simulink model "casper_sim_phase0"  (R2025b)
settings: Solver=FixedStepDiscrete  StartTime=-5  StopTime=5  FixedStep=1e-3  RelTol=1e-3
InitFcn:
  | casper_prelaunch_pad_truth_ts(5.0);
undefined symbols (not defined in the file or in its folder): Estimator
libraries: imu_block_visual x2, baro_block_visual x1, gps_block_visual x1, mag_block_visual x1
settings Model: Creator=Ashwin  LastModifiedBy=Ashwin
settings DebuggingCC: InheritedTsInSrcMsg=none

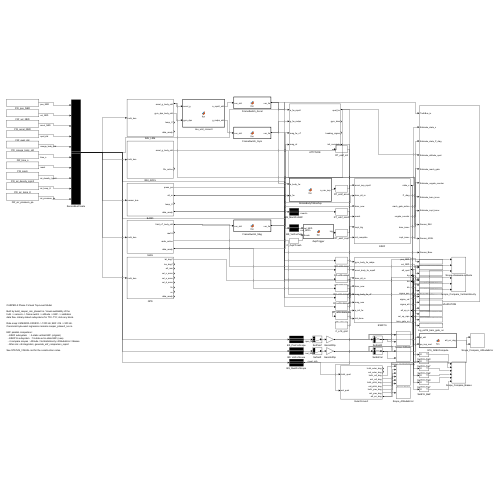
[thumbnail: Simulink's stored preview of the top-level diagram]
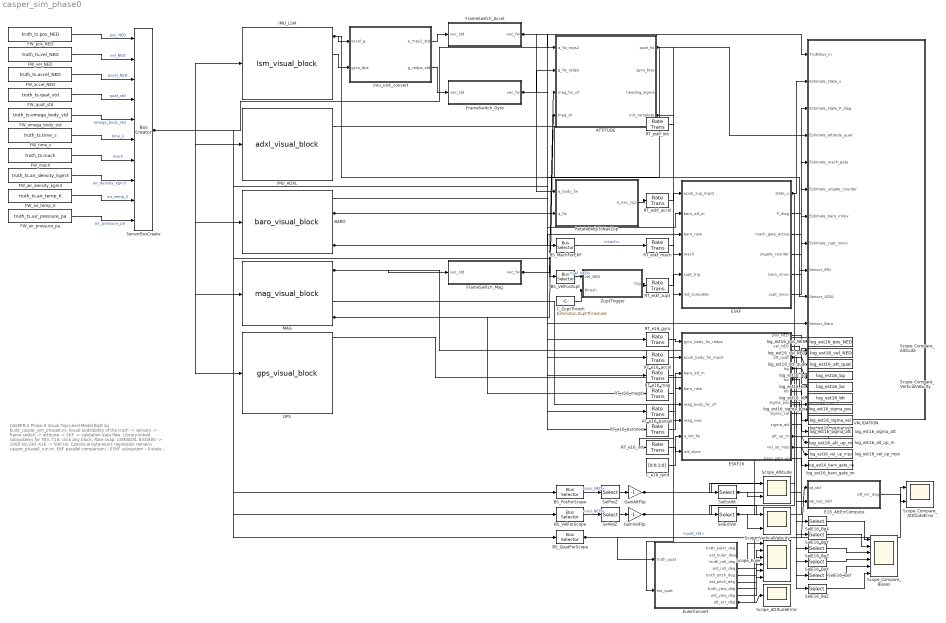
== system casper_sim_phase0 ==
  note: CASPER-2 Phase 0 Visual Top-Level Model
      |
      | Built by build_casper_sim_phase0.m. Visual auditability of the
      | truth -> sensors -> frame switch -> attitude -> EKF -> validation
      | data flow. Library-linked subsystems for T03..T10; click any block.
      |
      | Rate snap: LSM/ADXL 833/800 -> 1000 Hz; EKF 416 -> 500 Hz.
      | Canonical byte-exact regression remains casper_phase0_run.m.
      |
      | EKF parallel comparison:
      |   - ESKF subsystem    : 4-state vertical EKF (original)
      |   - ESKF16 subsystem  : 16-state error-state EKF (new)
      |   - 4 compare scopes  : Altitude / VerticalVelocity / AttitudeError / Biases
      |   - After sim: cd integration; generate_ekf_comparison_report
      |
      | See STATUS_VISUAL.md for the construction notes.
  ATTITUDE : Subsystem
  BARO : baro_block_visual/baro_visual_block  SystemSampleTime=-1  VariantActivationTime=update diagram  EmptyChoice=off  PassThrough=off  PassThroughVariantControl=(default)  EmptyChoiceVariantControl=(default)  AllowFlexibleInterface=on  Latency=0  AutoFrameSizeCalculation=off
  BS_MachForEKF : BusSelector  OutputSignals=mach
  BS_PosForScope : BusSelector  OutputSignals=pos_NED
  BS_QuatForScope : BusSelector  OutputSignals=quat_std
  BS_VelForScope : BusSelector  OutputSignals=vel_NED
  BS_VelForZupt : BusSelector  OutputSignals=vel_NED
  C_ZuptThresh : Constant  Value=Estimator.ZuptThreshold  SampleTime=-1
  C_e16_qinit : Constant  Value=[0;0;1;0]  SampleTime=-1
  E16_AttErrCompute : MATLAB Function  TreatAsAtomicUnit=on
  ESKF : Subsystem
  ESKF16 : Subsystem
  EulerConvert : Subsystem
  FW_accel_NED : FromWorkspace  VariableName=truth_ts.accel_NED  SampleTime=-1  ZeroCross=off  OutputAfterFinalValue=Holding final value
  FW_air_density_kgm3 : FromWorkspace  VariableName=truth_ts.air_density_kgm3  SampleTime=-1  ZeroCross=off  OutputAfterFinalValue=Holding final value
  FW_air_pressure_pa : FromWorkspace  VariableName=truth_ts.air_pressure_pa  SampleTime=-1  ZeroCross=off  OutputAfterFinalValue=Holding final value
  FW_air_temp_K : FromWorkspace  VariableName=truth_ts.air_temp_K  SampleTime=-1  ZeroCross=off  OutputAfterFinalValue=Holding final value
  FW_mach : FromWorkspace  VariableName=truth_ts.mach  SampleTime=-1  ZeroCross=off  OutputAfterFinalValue=Holding final value
  FW_omega_body_std : FromWorkspace  VariableName=truth_ts.omega_body_std  SampleTime=-1  ZeroCross=off  OutputAfterFinalValue=Holding final value
  FW_pos_NED : FromWorkspace  VariableName=truth_ts.pos_NED  SampleTime=-1  ZeroCross=off  OutputAfterFinalValue=Holding final value
  FW_quat_std : FromWorkspace  VariableName=truth_ts.quat_std  SampleTime=-1  ZeroCross=off  OutputAfterFinalValue=Holding final value
  FW_time_s : FromWorkspace  VariableName=truth_ts.time_s  SampleTime=-1  ZeroCross=off  OutputAfterFinalValue=Holding final value
  FW_vel_NED : FromWorkspace  VariableName=truth_ts.vel_NED  SampleTime=-1  ZeroCross=off  OutputAfterFinalValue=Holding final value
  FrameSwitch_Accel : MATLAB Function  TreatAsAtomicUnit=on
  FrameSwitch_Gyro : MATLAB Function  TreatAsAtomicUnit=on
  FrameSwitch_Mag : MATLAB Function  TreatAsAtomicUnit=on
  GPS : gps_block_visual/gps_visual_block  SystemSampleTime=-1  VariantActivationTime=update diagram  EmptyChoice=off  PassThrough=off  PassThroughVariantControl=(default)  EmptyChoiceVariantControl=(default)  AllowFlexibleInterface=on  Latency=0  AutoFrameSizeCalculation=off
  GainAltFlip : Gain  Gain=-1
  GainVelFlip : Gain  Gain=-1
  IMU_ADXL : imu_block_visual/adxl_visual_block  SystemSampleTime=-1  VariantActivationTime=update diagram  EmptyChoice=off  PassThrough=off  PassThroughVariantControl=(default)  EmptyChoiceVariantControl=(default)  AllowFlexibleInterface=on  Latency=0  AutoFrameSizeCalculation=off
  IMU_LSM : imu_block_visual/lsm_visual_block  SystemSampleTime=-1  VariantActivationTime=update diagram  EmptyChoice=off  PassThrough=off  PassThroughVariantControl=(default)  EmptyChoiceVariantControl=(default)  AllowFlexibleInterface=on  Latency=0  AutoFrameSizeCalculation=off
  MAG : mag_block_visual/mag_visual_block  SystemSampleTime=-1  VariantActivationTime=update diagram  EmptyChoice=off  PassThrough=off  PassThroughVariantControl=(default)  EmptyChoiceVariantControl=(default)  AllowFlexibleInterface=on  Latency=0  AutoFrameSizeCalculation=off
  RT_e16_accel : RateTransition  OutPortSampleTime=2e-3
  RT_e16_baroalt : RateTransition  OutPortSampleTime=2e-3
  RT_e16_baronew : RateTransition  OutPortSampleTime=2e-3
  RT_e16_gyro : RateTransition  OutPortSampleTime=2e-3
  RT_e16_init : RateTransition  OutPortSampleTime=2e-3
  RT_e16_mag : RateTransition  OutPortSampleTime=2e-3
  RT_e16_magdr : RateTransition  OutPortSampleTime=2e-3
  RT_eskf_accel : RateTransition  OutPortSampleTime=2e-3
  RT_eskf_init : RateTransition  OutPortSampleTime=2e-3
  RT_eskf_mach : RateTransition  OutPortSampleTime=2e-3
  RT_eskf_zupt : RateTransition  OutPortSampleTime=2e-3
  RotateBodyToNavZup : MATLAB Function  TreatAsAtomicUnit=on
  Scope_Altitude : Scope  NumInputPorts=2
      settings: Title=Altitude - truth vs estimate [m]
  Scope_AttitudeError : Scope
      settings: Title=Attitude error magnitude [deg]
  Scope_Compare_Altitude : Scope  NumInputPorts=3
      settings: Title=Altitude compare - truth vs 4-state vs 16-state [m]
  Scope_Compare_AttitudeError : Scope  NumInputPorts=2
      settings: Title=Attitude error compare - 4-state vs 16-state [deg]
  Scope_Compare_Biases : Scope  NumInputPorts=6
      settings: Title=16-state biases - gyro xyz (rad/s) + accel xyz (m/s^2)
  Scope_Compare_VerticalVelocity : Scope  NumInputPorts=3
      settings: Title=Vertical velocity compare - truth vs 4-state vs 16-state [m/s]
  Scope_Euler : Scope  NumInputPorts=6
      settings: Title=Orientation Euler - truth vs estimate [deg]
  Scope_VerticalVelocity : Scope  NumInputPorts=2
      settings: Title=Vertical velocity - truth vs estimate [m/s]
  SelE16_BaX : Selector  InputPortWidth=3  IndexOptions=Index vector (dialog)  Indices=1  OutputSizes=1
  SelE16_BaY : Selector  InputPortWidth=3  IndexOptions=Index vector (dialog)  Indices=2  OutputSizes=1
  SelE16_BaZ : Selector  InputPortWidth=3  IndexOptions=Index vector (dialog)  Indices=3  OutputSizes=1
  SelE16_BgX : Selector  InputPortWidth=3  IndexOptions=Index vector (dialog)  Indices=1  OutputSizes=1
  SelE16_BgY : Selector  InputPortWidth=3  IndexOptions=Index vector (dialog)  Indices=2  OutputSizes=1
  SelE16_BgZ : Selector  InputPortWidth=3  IndexOptions=Index vector (dialog)  Indices=3  OutputSizes=1
  SelEstAlt : Selector  InputPortWidth=4  IndexOptions=Index vector (dialog)  Indices=1  OutputSizes=1
  SelEstVel : Selector  InputPortWidth=4  IndexOptions=Index vector (dialog)  Indices=2  OutputSizes=1
  SelPosZ : Selector  InputPortWidth=3  IndexOptions=Index vector (dialog)  Indices=3  OutputSizes=1
  SelVelZ : Selector  InputPortWidth=3  IndexOptions=Index vector (dialog)  Indices=3  OutputSizes=1
  SensorBusCreate : BusCreator  Inputs=10  OutDataTypeStr=Bus: SensorInputBus  NonVirtualBus=on
  VALIDATION : Subsystem
  ZuptTrigger : MATLAB Function  TreatAsAtomicUnit=on
  imu_unit_convert : MATLAB Function  TreatAsAtomicUnit=on
  log_est16_alt_up_m : ToWorkspace  VariableName=log_est16_alt_up_m  SaveFormat=Structure With Time  SampleTime=-1
  log_est16_att_quat : ToWorkspace  VariableName=log_est16_att_quat  SaveFormat=Structure With Time  SampleTime=-1
  log_est16_ba : ToWorkspace  VariableName=log_est16_ba  SaveFormat=Structure With Time  SampleTime=-1
  log_est16_baro_gate_on : ToWorkspace  VariableName=log_est16_baro_gate_on  SaveFormat=Structure With Time  SampleTime=-1
  log_est16_bb : ToWorkspace  VariableName=log_est16_bb  SaveFormat=Structure With Time  SampleTime=-1
  log_est16_bg : ToWorkspace  VariableName=log_est16_bg  SaveFormat=Structure With Time  SampleTime=-1
  log_est16_pos_NED : ToWorkspace  VariableName=log_est16_pos_NED  SaveFormat=Structure With Time  SampleTime=-1
  log_est16_sigma_att : ToWorkspace  VariableName=log_est16_sigma_att  SaveFormat=Structure With Time  SampleTime=-1
  log_est16_sigma_pos : ToWorkspace  VariableName=log_est16_sigma_pos  SaveFormat=Structure With Time  SampleTime=-1
  log_est16_sigma_vel : ToWorkspace  VariableName=log_est16_sigma_vel  SaveFormat=Structure With Time  SampleTime=-1
  log_est16_vel_NED : ToWorkspace  VariableName=log_est16_vel_NED  SaveFormat=Structure With Time  SampleTime=-1
  log_est16_vel_up_mps : ToWorkspace  VariableName=log_est16_vel_up_mps  SaveFormat=Structure With Time  SampleTime=-1
  wires:
  FW_pos_NED/1 -> SensorBusCreate/1  "pos_NED"
  FW_vel_NED/1 -> SensorBusCreate/2  "vel_NED"
  FW_accel_NED/1 -> SensorBusCreate/3  "accel_NED"
  FW_quat_std/1 -> SensorBusCreate/4  "quat_std"
  FW_omega_body_std/1 -> SensorBusCreate/5  "omega_body_std"
  FW_time_s/1 -> SensorBusCreate/6  "time_s"
  FW_mach/1 -> SensorBusCreate/7  "mach"
  FW_air_density_kgm3/1 -> SensorBusCreate/8  "air_density_kgm3"
  FW_air_temp_K/1 -> SensorBusCreate/9  "air_temp_K"
  FW_air_pressure_pa/1 -> SensorBusCreate/10  "air_pressure_pa"
  SensorBusCreate/1 -> IMU_LSM/1, IMU_ADXL/1, BARO/1, MAG/1, GPS/1, BS_MachForEKF/1, BS_VelForZupt/1, VALIDATION/1(TruthBus_in), BS_PosForScope/1, BS_VelForScope/1, BS_QuatForScope/1
  IMU_LSM/1 -> imu_unit_convert/1(accel_g), VALIDATION/9(Sensor_IMU)
  IMU_LSM/2 -> imu_unit_convert/2(gyro_dps)
  imu_unit_convert/1(a_mps2_std) -> FrameSwitch_Accel/1(vec_std)
  imu_unit_convert/2(g_radps_std) -> FrameSwitch_Gyro/1(vec_std)
  MAG/1 -> FrameSwitch_Mag/1(vec_std), VALIDATION/12(Sensor_Mag)
  FrameSwitch_Accel/1(vec_fw) -> ATTITUDE/1(a_fw_mps2), RotateBodyToNavZup/1(a_body_fw), RT_e16_accel/1
  FrameSwitch_Gyro/1(vec_fw) -> ATTITUDE/2(g_fw_radps), RT_e16_gyro/1
  FrameSwitch_Mag/1(vec_fw) -> ATTITUDE/3(mag_fw_uT), RT_e16_mag/1
  MAG/4 -> ATTITUDE/4(mag_dr), RT_e16_magdr/1
  ATTITUDE/1(quat_fw) -> RotateBodyToNavZup/2(q_fw), VALIDATION/4(Estimate_attitude_quat), EulerConvert/2(est_quat)
  RotateBodyToNavZup/1(a_nav_zup) -> RT_eskf_accel/1
  BS_MachForEKF/1 -> RT_eskf_mach/1  "<mach>"
  BS_VelForZupt/1 -> ZuptTrigger/1(vel_NED)  "<vel_NED>"
  C_ZuptThresh/1 -> ZuptTrigger/2(thresh)
  ZuptTrigger/1(trig) -> RT_eskf_zupt/1
  ATTITUDE/4(init_complete) -> RT_eskf_init/1, RT_e16_init/1
  RT_eskf_accel/1 -> ESKF/1(accel_zup_mps2)
  BARO/2 -> ESKF/2(baro_alt_m), RT_e16_baroalt/1
  BARO/4 -> ESKF/3(baro_new), RT_e16_baronew/1
  RT_eskf_mach/1 -> ESKF/4(mach)
  RT_eskf_zupt/1 -> ESKF/5(zupt_trig)
  RT_eskf_init/1 -> ESKF/6(init_complete)
  ESKF/1(state_x) -> VALIDATION/2(Estimate_state_x), SelEstAlt/1, SelEstVel/1
  ESKF/2(P_diag) -> VALIDATION/3(Estimate_state_P_diag)
  ESKF/3(mach_gate_active) -> VALIDATION/5(Estimate_mach_gate)
  ESKF/4(ungate_counter) -> VALIDATION/6(Estimate_ungate_counter)
  ESKF/5(baro_innov) -> VALIDATION/7(Estimate_baro_innov)
  ESKF/6(zupt_innov) -> VALIDATION/8(Estimate_zupt_innov)
  IMU_ADXL/1 -> VALIDATION/10(Sensor_ADXL)
  BARO/1 -> VALIDATION/11(Sensor_Baro)
  GPS/1 -> VALIDATION/13(Sensor_GPS)
  MAG/3 -> VALIDATION/14(RadioTX_active)
  BS_PosForScope/1 -> SelPosZ/1  "<pos_NED>"
  SelPosZ/1 -> GainAltFlip/1
  BS_VelForScope/1 -> SelVelZ/1  "<vel_NED>"
  SelVelZ/1 -> GainVelFlip/1
  BS_QuatForScope/1 -> EulerConvert/1(truth_quat), E16_AttErrCompute/1(qt_std)  "<quat_std>"
  GainAltFlip/1 -> Scope_Altitude/1, Scope_Compare_Altitude/1
  SelEstAlt/1 -> Scope_Altitude/2, Scope_Compare_Altitude/2
  GainVelFlip/1 -> Scope_VerticalVelocity/1, Scope_Compare_VerticalVelocity/1
  SelEstVel/1 -> Scope_VerticalVelocity/2, Scope_Compare_VerticalVelocity/2
  EulerConvert/3(truth_roll_deg) -> Scope_Euler/1
  EulerConvert/4(est_roll_deg) -> Scope_Euler/2
  EulerConvert/5(truth_pitch_deg) -> Scope_Euler/3
  EulerConvert/6(est_pitch_deg) -> Scope_Euler/4
  EulerConvert/7(truth_yaw_deg) -> Scope_Euler/5
  EulerConvert/8(est_yaw_deg) -> Scope_Euler/6
  EulerConvert/9(att_err_deg) -> Scope_AttitudeError/1, Scope_Compare_AttitudeError/1
  RT_e16_gyro/1 -> ESKF16/1(gyro_body_fw_radps)
  RT_e16_accel/1 -> ESKF16/2(accel_body_fw_mps2)
  RT_e16_baroalt/1 -> ESKF16/3(baro_alt_m)
  RT_e16_baronew/1 -> ESKF16/4(baro_new)
  RT_e16_mag/1 -> ESKF16/5(mag_body_fw_uT)
  RT_e16_magdr/1 -> ESKF16/6(mag_new)
  C_e16_qinit/1 -> ESKF16/7(q_init_fw)
  RT_e16_init/1 -> ESKF16/8(init_done)
  ESKF16/1(pos_NED) -> log_est16_pos_NED/1
  ESKF16/2(vel_NED) -> log_est16_vel_NED/1
  ESKF16/3(att_quat) -> log_est16_att_quat/1, E16_AttErrCompute/2(qe_zup_ned)
  ESKF16/4(bg) -> log_est16_bg/1, SelE16_BgX/1, SelE16_BgY/1, SelE16_BgZ/1
  ESKF16/5(ba) -> log_est16_ba/1, SelE16_BaX/1, SelE16_BaY/1, SelE16_BaZ/1
  ESKF16/6(bb) -> log_est16_bb/1
  ESKF16/7(sigma_pos) -> log_est16_sigma_pos/1
  ESKF16/8(sigma_vel) -> log_est16_sigma_vel/1
  ESKF16/9(sigma_att) -> log_est16_sigma_att/1
  ESKF16/10(alt_up_m) -> log_est16_alt_up_m/1, Scope_Compare_Altitude/3
  ESKF16/11(vel_up_mps) -> log_est16_vel_up_mps/1, Scope_Compare_VerticalVelocity/3
  ESKF16/12(baro_gate_on) -> log_est16_baro_gate_on/1
  E16_AttErrCompute/1(att_err_deg) -> Scope_Compare_AttitudeError/2
  SelE16_BgX/1 -> Scope_Compare_Biases/1
  SelE16_BgY/1 -> Scope_Compare_Biases/2
  SelE16_BgZ/1 -> Scope_Compare_Biases/3
  SelE16_BaX/1 -> Scope_Compare_Biases/4
  SelE16_BaY/1 -> Scope_Compare_Biases/5
  SelE16_BaZ/1 -> Scope_Compare_Biases/6

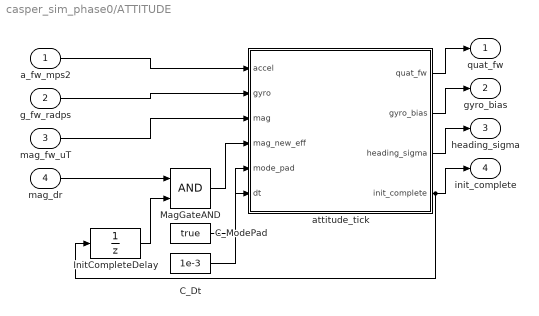
== system casper_sim_phase0/ATTITUDE ==
  a_fw_mps2 : Inport
  g_fw_radps : Inport  Port=2
  mag_fw_uT : Inport  Port=3
  mag_dr : Inport  Port=4
  C_Dt : Constant  Value=1e-3  SampleTime=-1
  C_ModePad : Constant  Value=true  OutDataTypeStr=boolean  SampleTime=-1
  InitCompleteDelay : UnitDelay  SampleTime=-1  HasFrameUpgradeWarning=on
  MagGateAND : Logic  AllPortsSameDT=off  OutDataTypeStr=boolean
  attitude_tick : MATLAB Function  TreatAsAtomicUnit=on
  quat_fw : Outport
  gyro_bias : Outport  Port=2
  heading_sigma : Outport  Port=3
  init_complete : Outport  Port=4
  wires:
  mag_dr/1 -> MagGateAND/1
  InitCompleteDelay/1 -> MagGateAND/2
  a_fw_mps2/1 -> attitude_tick/1(accel)
  g_fw_radps/1 -> attitude_tick/2(gyro)
  mag_fw_uT/1 -> attitude_tick/3(mag)
  MagGateAND/1 -> attitude_tick/4(mag_new_eff)
  C_ModePad/1 -> attitude_tick/5(mode_pad)
  C_Dt/1 -> attitude_tick/6(dt)
  attitude_tick/4(init_complete) -> InitCompleteDelay/1, init_complete/1
  attitude_tick/1(quat_fw) -> quat_fw/1
  attitude_tick/2(gyro_bias) -> gyro_bias/1
  attitude_tick/3(heading_sigma) -> heading_sigma/1

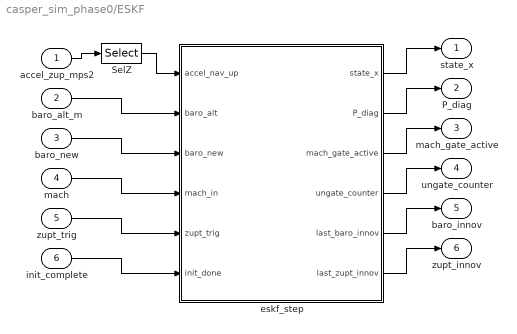
== system casper_sim_phase0/ESKF ==
  accel_zup_mps2 : Inport
  baro_alt_m : Inport  Port=2
  baro_new : Inport  Port=3
  mach : Inport  Port=4
  zupt_trig : Inport  Port=5
  init_complete : Inport  Port=6
  SelZ : Selector  InputPortWidth=3  IndexOptions=Index vector (dialog)  Indices=3  OutputSizes=1
  eskf_step : MATLAB Function  TreatAsAtomicUnit=on
  state_x : Outport
  P_diag : Outport  Port=2
  mach_gate_active : Outport  Port=3
  ungate_counter : Outport  Port=4
  baro_innov : Outport  Port=5
  zupt_innov : Outport  Port=6
  wires:
  accel_zup_mps2/1 -> SelZ/1
  SelZ/1 -> eskf_step/1(accel_nav_up)
  baro_alt_m/1 -> eskf_step/2(baro_alt)
  baro_new/1 -> eskf_step/3(baro_new)
  mach/1 -> eskf_step/4(mach_in)
  zupt_trig/1 -> eskf_step/5(zupt_trig)
  init_complete/1 -> eskf_step/6(init_done)
  eskf_step/1(state_x) -> state_x/1
  eskf_step/2(P_diag) -> P_diag/1
  eskf_step/3(mach_gate_active) -> mach_gate_active/1
  eskf_step/4(ungate_counter) -> ungate_counter/1
  eskf_step/5(last_baro_innov) -> baro_innov/1
  eskf_step/6(last_zupt_innov) -> zupt_innov/1

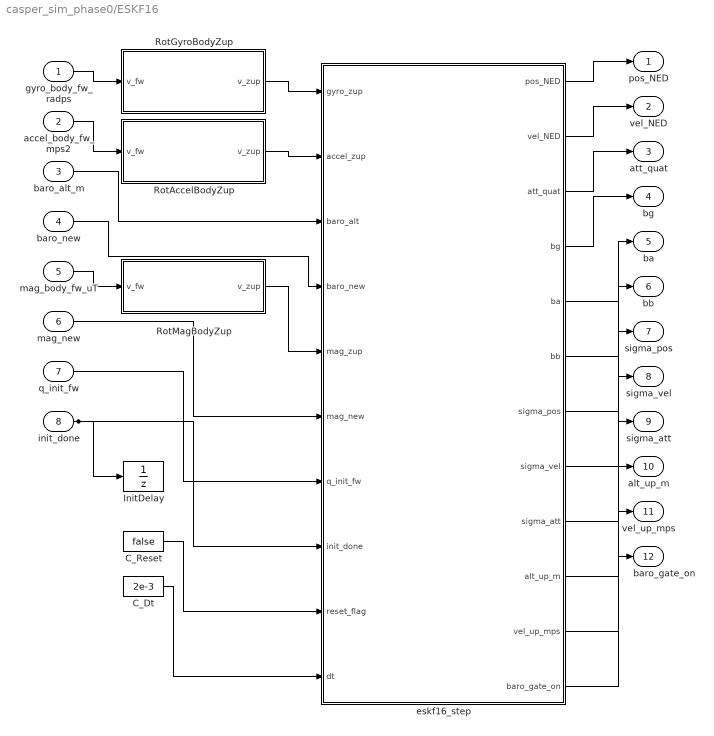
== system casper_sim_phase0/ESKF16 ==
  gyro_body_fw_radps : Inport
  accel_body_fw_mps2 : Inport  Port=2
  baro_alt_m : Inport  Port=3
  baro_new : Inport  Port=4
  mag_body_fw_uT : Inport  Port=5
  mag_new : Inport  Port=6
  q_init_fw : Inport  Port=7
  init_done : Inport  Port=8
  C_Dt : Constant  Value=2e-3  SampleTime=-1
  C_Reset : Constant  Value=false  OutDataTypeStr=boolean  SampleTime=-1
  InitDelay : UnitDelay  SampleTime=-1  HasFrameUpgradeWarning=on
  RotAccelBodyZup : MATLAB Function  TreatAsAtomicUnit=on
  RotGyroBodyZup : MATLAB Function  TreatAsAtomicUnit=on
  RotMagBodyZup : MATLAB Function  TreatAsAtomicUnit=on
  eskf16_step : MATLAB Function  TreatAsAtomicUnit=on
  pos_NED : Outport
  vel_NED : Outport  Port=2
  att_quat : Outport  Port=3
  bg : Outport  Port=4
  ba : Outport  Port=5
  bb : Outport  Port=6
  sigma_pos : Outport  Port=7
  sigma_vel : Outport  Port=8
  sigma_att : Outport  Port=9
  alt_up_m : Outport  Port=10
  vel_up_mps : Outport  Port=11
  baro_gate_on : Outport  Port=12
  wires:
  eskf16_step/12(baro_gate_on) -> baro_gate_on/1
  eskf16_step/11(vel_up_mps) -> vel_up_mps/1
  eskf16_step/10(alt_up_m) -> alt_up_m/1
  eskf16_step/9(sigma_att) -> sigma_att/1
  eskf16_step/8(sigma_vel) -> sigma_vel/1
  eskf16_step/7(sigma_pos) -> sigma_pos/1
  eskf16_step/6(bb) -> bb/1
  eskf16_step/5(ba) -> ba/1
  eskf16_step/4(bg) -> bg/1
  eskf16_step/3(att_quat) -> att_quat/1
  eskf16_step/2(vel_NED) -> vel_NED/1
  eskf16_step/1(pos_NED) -> pos_NED/1
  C_Dt/1 -> eskf16_step/10(dt)
  C_Reset/1 -> eskf16_step/9(reset_flag)
  q_init_fw/1 -> eskf16_step/7(q_init_fw)
  mag_new/1 -> eskf16_step/6(mag_new)
  RotMagBodyZup/1(v_zup) -> eskf16_step/5(mag_zup)
  baro_new/1 -> eskf16_step/4(baro_new)
  baro_alt_m/1 -> eskf16_step/3(baro_alt)
  RotAccelBodyZup/1(v_zup) -> eskf16_step/2(accel_zup)
  RotGyroBodyZup/1(v_zup) -> eskf16_step/1(gyro_zup)
  init_done/1 -> eskf16_step/8(init_done), InitDelay/1
  mag_body_fw_uT/1 -> RotMagBodyZup/1(v_fw)
  accel_body_fw_mps2/1 -> RotAccelBodyZup/1(v_fw)
  gyro_body_fw_radps/1 -> RotGyroBodyZup/1(v_fw)

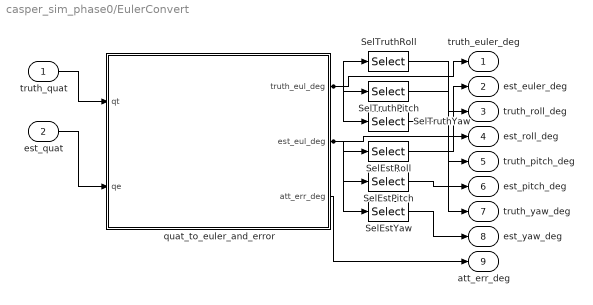
== system casper_sim_phase0/EulerConvert ==
  truth_quat : Inport
  est_quat : Inport  Port=2
  SelEstPitch : Selector  InputPortWidth=3  IndexOptions=Index vector (dialog)  Indices=2  OutputSizes=1
  SelEstRoll : Selector  InputPortWidth=3  IndexOptions=Index vector (dialog)  Indices=1  OutputSizes=1
  SelEstYaw : Selector  InputPortWidth=3  IndexOptions=Index vector (dialog)  Indices=3  OutputSizes=1
  SelTruthPitch : Selector  InputPortWidth=3  IndexOptions=Index vector (dialog)  Indices=2  OutputSizes=1
  SelTruthRoll : Selector  InputPortWidth=3  IndexOptions=Index vector (dialog)  Indices=1  OutputSizes=1
  SelTruthYaw : Selector  InputPortWidth=3  IndexOptions=Index vector (dialog)  Indices=3  OutputSizes=1
  quat_to_euler_and_error : MATLAB Function  TreatAsAtomicUnit=on
  truth_euler_deg : Outport
  est_euler_deg : Outport  Port=2
  truth_roll_deg : Outport  Port=3
  est_roll_deg : Outport  Port=4
  truth_pitch_deg : Outport  Port=5
  est_pitch_deg : Outport  Port=6
  truth_yaw_deg : Outport  Port=7
  est_yaw_deg : Outport  Port=8
  att_err_deg : Outport  Port=9
  wires:
  truth_quat/1 -> quat_to_euler_and_error/1(qt)
  est_quat/1 -> quat_to_euler_and_error/2(qe)
  quat_to_euler_and_error/1(truth_eul_deg) -> SelTruthRoll/1, SelTruthPitch/1, SelTruthYaw/1, truth_euler_deg/1
  quat_to_euler_and_error/2(est_eul_deg) -> SelEstRoll/1, SelEstPitch/1, SelEstYaw/1, est_euler_deg/1
  SelTruthRoll/1 -> truth_roll_deg/1
  SelEstRoll/1 -> est_roll_deg/1
  SelTruthPitch/1 -> truth_pitch_deg/1
  SelEstPitch/1 -> est_pitch_deg/1
  SelTruthYaw/1 -> truth_yaw_deg/1
  SelEstYaw/1 -> est_yaw_deg/1
  quat_to_euler_and_error/3(att_err_deg) -> att_err_deg/1

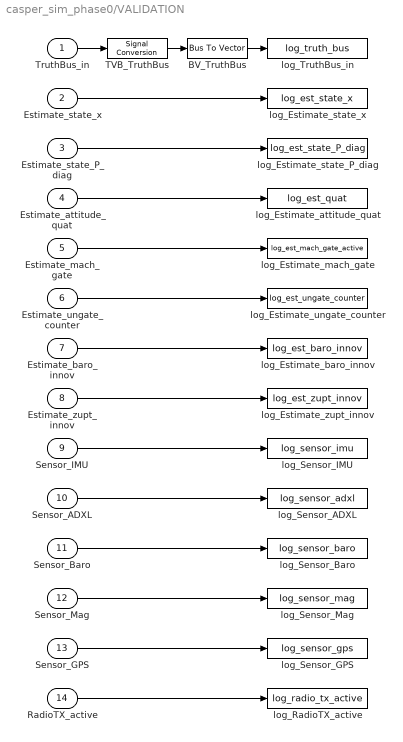
== system casper_sim_phase0/VALIDATION ==
  TruthBus_in : Inport
  Estimate_state_x : Inport  Port=2
  Estimate_state_P_diag : Inport  Port=3
  Estimate_attitude_quat : Inport  Port=4
  Estimate_mach_gate : Inport  Port=5
  Estimate_ungate_counter : Inport  Port=6
  Estimate_baro_innov : Inport  Port=7
  Estimate_zupt_innov : Inport  Port=8
  Sensor_IMU : Inport  Port=9
  Sensor_ADXL : Inport  Port=10
  Sensor_Baro : Inport  Port=11
  Sensor_Mag : Inport  Port=12
  Sensor_GPS : Inport  Port=13
  RadioTX_active : Inport  Port=14
  BV_TruthBus : BusToVector
  TVB_TruthBus : SignalConversion  ConversionOutput=Virtual bus  OverrideOpt=off
  log_Estimate_attitude_quat : ToWorkspace  VariableName=log_est_quat  SaveFormat=Structure With Time  SampleTime=-1
  log_Estimate_baro_innov : ToWorkspace  VariableName=log_est_baro_innov  SaveFormat=Structure With Time  SampleTime=-1
  log_Estimate_mach_gate : ToWorkspace  VariableName=log_est_mach_gate_active  SaveFormat=Structure With Time  SampleTime=-1
  log_Estimate_state_P_diag : ToWorkspace  VariableName=log_est_state_P_diag  SaveFormat=Structure With Time  SampleTime=-1
  log_Estimate_state_x : ToWorkspace  VariableName=log_est_state_x  SaveFormat=Structure With Time  SampleTime=-1
  log_Estimate_ungate_counter : ToWorkspace  VariableName=log_est_ungate_counter  SaveFormat=Structure With Time  SampleTime=-1
  log_Estimate_zupt_innov : ToWorkspace  VariableName=log_est_zupt_innov  SaveFormat=Structure With Time  SampleTime=-1
  log_RadioTX_active : ToWorkspace  VariableName=log_radio_tx_active  SaveFormat=Structure With Time  SampleTime=-1
  log_Sensor_ADXL : ToWorkspace  VariableName=log_sensor_adxl  SaveFormat=Structure With Time  SampleTime=-1
  log_Sensor_Baro : ToWorkspace  VariableName=log_sensor_baro  SaveFormat=Structure With Time  SampleTime=-1
  log_Sensor_GPS : ToWorkspace  VariableName=log_sensor_gps  SaveFormat=Structure With Time  SampleTime=-1
  log_Sensor_IMU : ToWorkspace  VariableName=log_sensor_imu  SaveFormat=Structure With Time  SampleTime=-1
  log_Sensor_Mag : ToWorkspace  VariableName=log_sensor_mag  SaveFormat=Structure With Time  SampleTime=-1
  log_TruthBus_in : ToWorkspace  VariableName=log_truth_bus  SaveFormat=Structure With Time  SampleTime=-1
  wires:
  TruthBus_in/1 -> TVB_TruthBus/1
  TVB_TruthBus/1 -> BV_TruthBus/1
  BV_TruthBus/1 -> log_TruthBus_in/1
  Estimate_state_x/1 -> log_Estimate_state_x/1
  Estimate_state_P_diag/1 -> log_Estimate_state_P_diag/1
  Estimate_attitude_quat/1 -> log_Estimate_attitude_quat/1
  Estimate_mach_gate/1 -> log_Estimate_mach_gate/1
  Estimate_ungate_counter/1 -> log_Estimate_ungate_counter/1
  Estimate_baro_innov/1 -> log_Estimate_baro_innov/1
  Estimate_zupt_innov/1 -> log_Estimate_zupt_innov/1
  Sensor_IMU/1 -> log_Sensor_IMU/1
  Sensor_ADXL/1 -> log_Sensor_ADXL/1
  Sensor_Baro/1 -> log_Sensor_Baro/1
  Sensor_Mag/1 -> log_Sensor_Mag/1
  Sensor_GPS/1 -> log_Sensor_GPS/1
  RadioTX_active/1 -> log_RadioTX_active/1

== matlab function casper_sim_phase0/EulerConvert/quat_to_euler_and_error ==
  data: qt input; truth_eul_deg output; qe input; est_eul_deg output; att_err_deg output
function [truth_eul_deg, est_eul_deg, att_err_deg] = fcn(qt, qe)
%#codegen
% Hamilton scalar-first quaternion -> Euler (ZYX: roll,pitch,yaw) in deg.
% Also computes magnitude of quat angle diff in deg.
%
% IMPORTANT FRAME NOTE:
%   qt (truth_quat) arrives in std-aircraft body -> NED-down convention
%     (X-fwd, Z-down). This is the convention RasAero / casper_truth_resample
%     emits via TruthBus.quat_std.
%   qe (est_quat) is in firmware body -> firmware nav (Y-nose, Z-up)
%     convention, as produced by casper_attitude_tick.
%
%   Comparing the two quats DIRECTLY (without frame switching truth) gives
%   a 90-180 deg "error" purely from the convention mismatch -- even when
%   the estimator is perfect. We therefore convert qt -> qt_fw using the
%   exact T_nav_quat * C_std * R_body' composition that
%   casper_frame_switch_quat() applies. Both factors are proper rotations
%   (det=+1) so the DCM round-trips cleanly through quaternion form.
qt = double(qt(:));
qe = double(qe(:));
nt = sqrt(qt(1)^2+qt(2)^2+qt(3)^2+qt(4)^2);
ne = sqrt(qe(1)^2+qe(2)^2+qe(3)^2+qe(4)^2);
if nt < 1e-12; nt = 1; end
if ne < 1e-12; ne = 1; end
qt = qt / nt;
qe = qe / ne;
% --- Frame switch: qt (std) -> qt_fw (firmware) ---
qt_fw = quat_std_to_fw_(qt);
% --- Euler (ZYX) from Hamilton [w x y z] ---
% Display the truth Euler in firmware-frame too so the Euler scope
% lines up with the estimator output channel-for-channel.
truth_eul_deg = quat_to_eul_zyx_(qt_fw) * (180/pi);
est_eul_deg   = quat_to_eul_zyx_(qe)    * (180/pi);
% --- Quat angle diff: q_err = qt_fw^-1 * qe, angle = 2*acos(|w|) ---
% Conjugate of unit quat = inverse.
qt_fw_inv = [qt_fw(1); -qt_fw(2); -qt_fw(3); -qt_fw(4)];
qe_q      = quat_mul_(qt_fw_inv, qe);
w_abs     = min(1.0, abs(qe_q(1)));
att_err_deg = 2 * acos(w_abs) * (180/pi);
end

function q_fw = quat_std_to_fw_(q_std)
%#codegen
% std-body-to-NED quat -> firmware-body-to-Zup quat. Mirrors
% casper_frame_switch_quat(): C_fw = T_nav_quat * C_std * R_body'.
C_std = dcm_from_quat_(q_std);
R_body     = [ 0 1 0; 1 0 0; 0 0 -1 ];
T_nav_quat = [ 0 1 0; 1 0 0; 0 0 -1 ];
C_fw = T_nav_quat * C_std * R_body.';
q_fw = quat_from_dcm_(C_fw);
if q_fw(1) < 0; q_fw = -q_fw; end
end

function C = dcm_from_quat_(q)
%#codegen
w = q(1); x = q(2); y = q(3); z = q(4);
C = [ 1 - 2*(y*y + z*z),  2*(x*y - z*w),       2*(x*z + y*w);
      2*(x*y + z*w),      1 - 2*(x*x + z*z),   2*(y*z - x*w);
      2*(x*z - y*w),      2*(y*z + x*w),       1 - 2*(x*x + y*y) ];
end

function q = quat_from_dcm_(C)
%#codegen
% Shepperd's algorithm. Mirrors casper_frame_switch_quat local_quat_from_dcm.
tr = C(1,1) + C(2,2) + C(3,3);
qw = 0; qx = 0; qy = 0; qz = 0;
if tr > 0
    s = sqrt(tr + 1.0) * 2.0;
    qw = 0.25 * s;
    qx = (C(3,2) - C(2,3)) / s;
    qy = (C(1,3) - C(3,1)) / s;
    qz = (C(2,1) - C(1,2)) / s;
elseif (C(1,1) > C(2,2)) && (C(1,1) > C(3,3))
    s = sqrt(1.0 + C(1,1) - C(2,2) - C(3,3)) * 2.0;
    qw = (C(3,2) - C(2,3)) / s;
    qx = 0.25 * s;
    qy = (C(1,2) + C(2,1)) / s;
    qz = (C(1,3) + C(3,1)) / s;
elseif C(2,2) > C(3,3)
    s = sqrt(1.0 + C(2,2) - C(1,1) - C(3,3)) * 2.0;
    qw = (C(1,3) - C(3,1)) / s;
    qx = (C(1,2) + C(2,1)) / s;
    qy = 0.25 * s;
    qz = (C(2,3) + C(3,2)) / s;
else
    s = sqrt(1.0 + C(3,3) - C(1,1) - C(2,2)) * 2.0;
    qw = (C(2,1) - C(1,2)) / s;
    qx = (C(1,3) + C(3,1)) / s;
    qy = (C(2,3) + C(3,2)) / s;
    qz = 0.25 * s;
end
q = [qw; qx; qy; qz];
n = sqrt(q(1)^2 + q(2)^2 + q(3)^2 + q(4)^2);
if n > 0; q = q / n; end
end

function eul = quat_to_eul_zyx_(q)
%#codegen
% q = [w x y z]; eul = [roll; pitch; yaw] (rad), ZYX intrinsic convention.
w = q(1); x = q(2); y = q(3); z = q(4);
% Roll (x-axis rotation)
sinr_cosp = 2 * (w*x + y*z);
cosr_cosp = 1 - 2 * (x*x + y*y);
roll  = atan2(sinr_cosp, cosr_cosp);
% Pitch (y-axis rotation), clamp for safety near +/-90deg
sinp = 2 * (w*y - z*x);
if sinp >  1; sinp =  1; end
if sinp < -1; sinp = -1; end
pitch = asin(sinp);
% Yaw (z-axis rotation)
siny_cosp = 2 * (w*z + x*y);
cosy_cosp = 1 - 2 * (y*y + z*z);
yaw   = atan2(siny_cosp, cosy_cosp);
eul = [roll; pitch; yaw];
end

function qo = quat_mul_(a, b)
%#codegen
% Hamilton quaternion product, scalar-first.
aw = a(1); ax = a(2); ay = a(3); az = a(4);
bw = b(1); bx = b(2); by = b(3); bz = b(4);
qo = [ aw*bw - ax*bx - ay*by - az*bz;
       aw*bx + ax*bw + ay*bz - az*by;
       aw*by - ax*bz + ay*bw + az*bx;
       aw*bz + ax*by - ay*bx + az*bw ];
end

== matlab function casper_sim_phase0/ESKF16/RotAccelBodyZup ==
  data: v_fw input; v_zup output
function v_zup = fcn(v_fw)
%#codegen
v_zup = double(v_fw(:));
end

== matlab function casper_sim_phase0/ESKF16/RotGyroBodyZup ==
  data: v_fw input; v_zup output
function v_zup = fcn(v_fw)
%#codegen
v_zup = double(v_fw(:));
end

== matlab function casper_sim_phase0/ESKF16/RotMagBodyZup ==
  data: v_fw input; v_zup output
function v_zup = fcn(v_fw)
%#codegen
v_zup = double(v_fw(:));
end

== matlab function casper_sim_phase0/ESKF16/eskf16_step ==
  data: gyro_zup input; pos_NED output; accel_zup input; baro_alt input; baro_new input; mag_zup input; mag_new input; q_init_fw input; init_done input; reset_flag input; dt input; vel_NED output; att_quat output; bg output; ba output; bb output; sigma_pos output; sigma_vel output; sigma_att output; alt_up_m output; vel_up_mps output; baro_gate_on output
function [pos_NED, vel_NED, att_quat, bg, ba, bb, sigma_pos, sigma_vel, sigma_att, alt_up_m, vel_up_mps, baro_gate_on] = fcn(gyro_zup, accel_zup, baro_alt, baro_new, mag_zup, mag_new, q_init_fw, init_done, reset_flag, dt)
%#codegen
coder.extrinsic('casper_eskf16_helper');
pos_NED      = zeros(3,1);
vel_NED      = zeros(3,1);
att_quat     = [0;0;1;0];
bg           = zeros(3,1);
ba           = zeros(3,1);
bb           = double(0);
sigma_pos    = zeros(3,1);
sigma_vel    = zeros(3,1);
sigma_att    = zeros(3,1);
alt_up_m     = double(0);
vel_up_mps   = double(0);
baro_gate_on = false;
baro_innov_unused = double(0);
init_armed_unused = false;
[pos_NED, vel_NED, att_quat, bg, ba, bb, sigma_pos, sigma_vel, sigma_att, baro_gate_on, baro_innov_unused, init_armed_unused] = casper_eskf16_helper(double(gyro_zup), double(accel_zup), double(baro_alt), logical(baro_new), double(mag_zup), logical(mag_new), double(q_init_fw), logical(init_done), logical(reset_flag), double(dt));
alt_up_m   = -double(pos_NED(3));
vel_up_mps = -double(vel_NED(3));
end

== matlab function casper_sim_phase0/E16_AttErrCompute ==
  data: qt_std input; att_err_deg output; qe_zup_ned input
function att_err_deg = fcn(qt_std, qe_zup_ned)
%#codegen
qt = double(qt_std(:));
qe = double(qe_zup_ned(:));
nt = sqrt(qt(1)^2+qt(2)^2+qt(3)^2+qt(4)^2);
ne = sqrt(qe(1)^2+qe(2)^2+qe(3)^2+qe(4)^2);
if nt < 1e-12; nt = 1; end
if ne < 1e-12; ne = 1; end
qt = qt / nt;
qe = qe / ne;
% q_err = qt^-1 * qe  -> angle = 2*acos(|w|)
qt_inv = [qt(1); -qt(2); -qt(3); -qt(4)];
aw = qt_inv(1); ax = qt_inv(2); ay = qt_inv(3); az = qt_inv(4);
bw = qe(1);     bx = qe(2);     by = qe(3);     bz = qe(4);
w  = aw*bw - ax*bx - ay*by - az*bz;
w_abs = min(1.0, abs(w));
att_err_deg = 2 * acos(w_abs) * (180/pi);
end

== matlab function casper_sim_phase0/FrameSwitch_Accel ==
  data: vec_std input; vec_fw output
function vec_fw = fcn(vec_std)
%#codegen
v = double(vec_std(:));
vec_fw = [ v(2); v(1); -v(3) ];
end

== matlab function casper_sim_phase0/imu_unit_convert ==
  data: accel_g input; a_mps2_std output; gyro_dps input; g_radps_std output
function [a_mps2_std, g_radps_std] = fcn(accel_g, gyro_dps)
%#codegen
% Sign-flip: convert imuSensor industry convention (+ g UP on pad)
% to the legacy casper_imu_lsm_model convention (a_specific = a-g).
a_mps2_std  = -double(accel_g(:)) * 9.80665;
g_radps_std =  double(gyro_dps(:)) * (pi/180);
end

== matlab function casper_sim_phase0/FrameSwitch_Gyro ==
  data: vec_std input; vec_fw output
function vec_fw = fcn(vec_std)
%#codegen
v = double(vec_std(:));
vec_fw = [ v(2); v(1); -v(3) ];
end

== matlab function casper_sim_phase0/FrameSwitch_Mag ==
  data: vec_std input; vec_fw output
function vec_fw = fcn(vec_std)
%#codegen
v = double(vec_std(:));
vec_fw = [ v(2); v(1); -v(3) ];
end

== matlab function casper_sim_phase0/ATTITUDE/attitude_tick ==
  data: accel input; quat_fw output; gyro input; mag input; mag_new_eff input; mode_pad input; dt input; gyro_bias output; heading_sigma output; init_complete output
function [quat_fw, gyro_bias, heading_sigma, init_complete] = fcn(accel, gyro, mag, mag_new_eff, mode_pad, dt)
%#codegen
coder.extrinsic('attitude_step_helper');
% Preallocate outputs so chart parser can infer types.
quat_fw       = [1;0;0;0];
gyro_bias     = zeros(3,1);
heading_sigma = double(0);
init_complete = false;
[quat_fw, gyro_bias, heading_sigma, init_complete] = attitude_step_helper(double(accel), double(gyro), double(mag), logical(mag_new_eff), logical(mode_pad), double(dt));
end

== matlab function casper_sim_phase0/ESKF/eskf_step ==
  data: accel_nav_up input; state_x output; baro_alt input; baro_new input; mach_in input; zupt_trig input; init_done input; P_diag output; mach_gate_active output; ungate_counter output; last_baro_innov output; last_zupt_innov output
function [state_x, P_diag, mach_gate_active, ungate_counter, last_baro_innov, last_zupt_innov] = fcn(accel_nav_up, baro_alt, baro_new, mach_in, zupt_trig, init_done)
%#codegen
coder.extrinsic('eskf_step_helper');
% All outputs preallocated to fixed sizes so the chart parser can
% statically infer types even with extrinsic call.
state_x = zeros(4,1);
P_diag  = zeros(4,1);
mach_gate_active = double(0);
ungate_counter   = double(0);
last_baro_innov  = double(0);
last_zupt_innov  = double(0);
[state_x, P_diag, mach_gate_active, ungate_counter, last_baro_innov, last_zupt_innov] = eskf_step_helper(double(accel_nav_up), double(baro_alt), logical(baro_new), double(mach_in), logical(zupt_trig), logical(init_done));
end

== matlab function casper_sim_phase0/RotateBodyToNavZup ==
  data: a_body_fw input; a_nav_zup output; q_fw input
function a_nav_zup = fcn(a_body_fw, q_fw)
%#codegen
q = double(q_fw(:));
a = double(a_body_fw(:));
nq = sqrt(q(1)*q(1)+q(2)*q(2)+q(3)*q(3)+q(4)*q(4));
if nq < 1e-12; nq = 1; end
q = q / nq;
w = q(1); x = q(2); y = q(3); z = q(4);
R = [1-2*(y*y+z*z),   2*(x*y - z*w),   2*(x*z + y*w);
     2*(x*y + z*w),   1-2*(x*x+z*z),   2*(y*z - x*w);
     2*(x*z - y*w),   2*(y*z + x*w),   1-2*(x*x+y*y)];
a_nav_zup = R * a;
end

== matlab function casper_sim_phase0/ZuptTrigger ==
  data: vel_NED input; trig output; thresh input
function trig = fcn(vel_NED, thresh)
%#codegen
v = double(vel_NED(:));
trig = sqrt(v(1)^2 + v(2)^2 + v(3)^2) < double(thresh);
end
